simulink model "TVC_2D"  (R2020b)
settings: Solver=VariableStepAuto  StartTime=0.0  StopTime=10.0  RelTol=1e-3
libraries: pid_lib x1, simulink x1, cstblocks x1
settings Model: Creator=mluser  LastModifiedBy=mluser

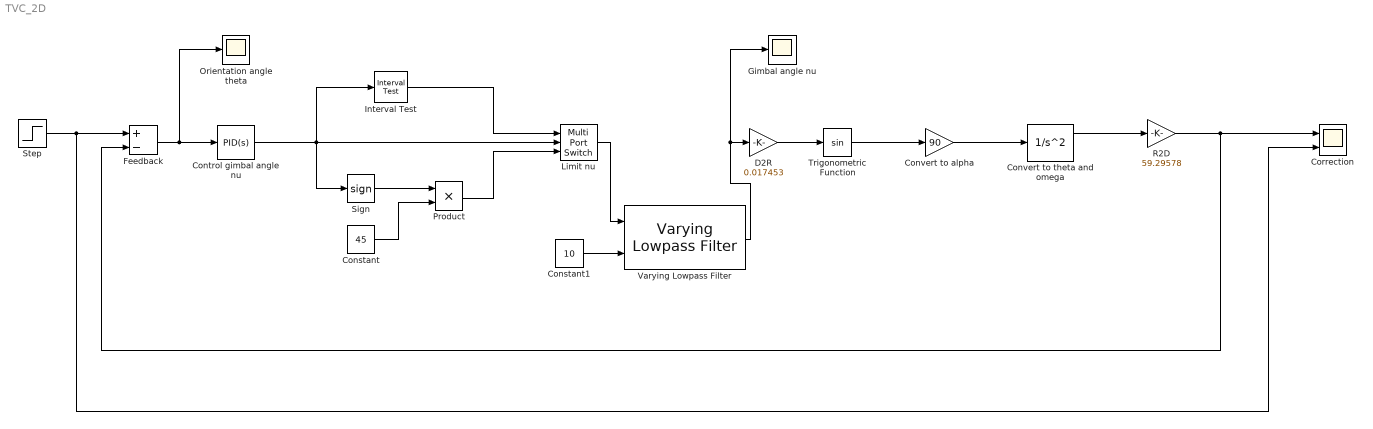
== system TVC_2D ==
  Constant : Constant  Value=45
  Constant1 : Constant  Value=10
  Control gimbal angle nu : pid_lib/PID Controller  Controller=PID  Form=Parallel  TimeDomain=Continuous-time  UseExternalTs=off  SampleTime=-1  IntegratorMethod=Forward Euler  FilterMethod=Forward Euler  ControllerParametersSource=internal  P=0.2  I=0.00047  D=0.06  UseFilter=on  N=100  TunerSelectOption=Transfer Function Based (PID Tuner App)  InitialConditionSource=internal  InitialConditionForIntegrator=0  InitialConditionForFilter=0  DifferentiatorICPrevScaledInput=0  ExternalReset=none  TrackingMode=off  Kt=1  LimitOutput=off  SatLimitsSource=internal  UpperSaturationLimit=inf  LowerSaturationLimit=-inf  LinearizeAsGain=on  AntiWindupMode=none  Kb=1  POutMin=[]  POutMax=[]  IOutMin=[]  IOutMax=[]  DOutMin=[]  DOutMax=[]  NOutMin=[]  NOutMax=[]  SumOutMin=[]  SumOutMax=[]  SaturationOutMin=[]  SaturationOutMax=[]  PParamMin=[]  PParamMax=[]  IParamMin=[]  IParamMax=[]  DParamMin=[]  DParamMax=[]  NParamMin=[]  NParamMax=[]  KbParamMin=[]  KbParamMax=[]  KtParamMin=[]  KtParamMax=[]  KbOutMin=[]  KbOutMax=[]  KtOutMin=[]  KtOutMax=[]  IntegratorOutMin=[]  IntegratorOutMax=[]  FilterOutMin=[]  FilterOutMax=[]  SumI1OutMin=[]  SumI1OutMax=[]  SumI2OutMin=[]  SumI2OutMax=[]  SumI3OutMin=[]  SumI3OutMax=[]  SumI4OutMin=[]  SumI4OutMax=[]  SumDOutMin=[]  SumDOutMax=[]  DifferentiatorOutMin=[]  DifferentiatorOutMax=[]  FilterDiffOutCoefMin=[]  FilterDiffOutCoefMax=[]  ReciprocalOutMin=[]  ReciprocalOutMax=[]  SumDenOutMin=[]  SumDenOutMax=[]  SumNumOutMin=[]  SumNumOutMax=[]  DivideOutMin=[]  DivideOutMax=[]  UdiffTsProdOutMin=[]  UdiffTsProdOutMax=[]  NTsProdOutMin=[]  NTsProdOutMax=[]  UintegralTsProdOutMin=[]  UintegralTsProdOutMax=[]  UngainTsProdOutMin=[]  UngainTsProdOutMax=[]  IntegratorContinuousStateAttributes=''  IntegratorStateMustResolveToSignalObject=off  IntegratorRTWStateStorageClass=Auto  FilterContinuousStateAttributes=''  FilterStateMustResolveToSignalObject=off  FilterRTWStateStorageClass=Auto  ParallelPVariant=InternalParameters  IdealPVariant=Disabled  IVariant=InternalParameters  DVariant=InternalParameters  IntegratorVariant=Continuous  SatVariant=Disabled  AWVariant=Passthrough  PCopyVariant=Disabled  TRVariant=Disabled  FdbkBlocksVariant=Forward  IdealPFdbkVariant=Disabled  SatFdbkVariant=Disabled  DerivativeFilterVariant=ContFilter  NVariant=InternalParameters  NCopyVariant=Disabled  FilterICVariant=InternalICsFilter  IntegratorICVariant=InternalICs  ExternalResetVariant=Disabled  TRSumVariant=Passthrough  SumFdbkVariant=Disabled  SumVariant=Sum_PID  TsampFilterVariant=InternalTs  TsampNgainVariant=Passthrough  TsampIntegralVariant=Passthrough  ExternalSaturationOutDataTypeStr=Inherit: Same as second input
  Convert to alpha : Gain  Gain=90
  Convert to theta and omega : SecondOrderIntegrator
  Correction : Scope  NumInputPorts=2
  D2R : Gain  Gain=0.017453
  Feedback : Sum  Inputs=+-
  Gimbal angle nu : Scope
  Interval Test : simulink/Logic and Bit Operations/Interval Test  IntervalClosedRight=on  uplimit=45  IntervalClosedLeft=on  lowlimit=-45  OutDataTypeStr=boolean
  Limit nu : MultiPortSwitch  DataPortOrder=Specify indices  Inputs=2  DataPortIndices={1,0}
  Orientation angle theta : Scope
  Product : Product
  R2D : Gain  Gain=59.29578
  Sign : Signum
  Step : Step  After=45  SampleTime=0
  Trigonometric Function : Trigonometry
  Varying Lowpass Filter : cstblocks/Linear Parameter Varying/Varying Lowpass Filter  N=1
  wires:
  Step/1 -> Feedback/1, Correction/2
  Feedback/1 -> Orientation angle theta/1, Control gimbal angle nu/1
  Convert to alpha/1 -> Convert to theta and omega/1
  D2R/1 -> Trigonometric Function/1
  Trigonometric Function/1 -> Convert to alpha/1
  Convert to theta and omega/1 -> R2D/1
  R2D/1 -> Correction/1, Feedback/2
  Control gimbal angle nu/1 -> Limit nu/2, Interval Test/1, Sign/1
  Interval Test/1 -> Limit nu/1
  Sign/1 -> Product/1
  Product/1 -> Limit nu/3
  Constant/1 -> Product/2
  Limit nu/1 -> Varying Lowpass Filter/1
  Varying Lowpass Filter/1 -> Gimbal angle nu/1, D2R/1
  Constant1/1 -> Varying Lowpass Filter/2
